simulink model "Working_TASS2_Fossen"  (Simulink 7.4)
settings: Solver=ode5  StartTime=0  StopTime=30  FixedStep=DeltaT  RelTol=1e-3
InitFcn:
  | %Bifocal Relay Mirror Spacecraft Dynamics Simulation          TA Sands
  | clear all;close all;clc;
  | 
  | %Constants0
  | Re=6371.2e3;mu=398601.2e9;          %earth radius and universal gravitation constant
  | 
  | %Spacecraft orbit
  | h=0;                                     %orbit altitude
  | R=Re+h;                             %orbit radius from center of earth
  | we=0.000072921158553;   %earth's angular velocity rad/solar sec(Vallado)
  | wo=sqrt(mu/(Re+h)^3);        %orbit angular velocity
  | incln=36.6001*pi/180;          %Inclination assumed Monterey Latitude
  | epsilon=12*pi/180;  alphao=0;
  | uo=0; nuo=0;                        %Start S/C beneath subsolar point
  | beta=60; gamma=1.5;
  | a=0.545491852; b=0.314939867;  c=0.704226952;   %Assumed spacecraft rectangular size
  | Area=[b*c a*c a*b];                 %projected area~m^2 in body x,y,z directions
  | density=4.39e-14;
  | kpre=-9.9639/24/3600/180*pi*0;      %nodal precession constant assumed zero here
  | wn=kpre*(Re/(Re+h))^3.5*cos(incln); %nodal precession (zero eccentricity)
  | V=wo*(Re+h);
  | rho=asin(Re/(h+Re));                %earth angular radius
  | Cd=2.5;     psun=4.5E-6;            %Drag coefficient and solar pressure constant~N/m^2
  | Kaero=-0.5*Cd*V^2;   Psolar=2*psun;  %constants for aero and solar torque calculation
  | dL=[0.002 0.002 0.008];             %predicted distance between cp and cg
  | Kme=2.3390e-005;
  | 
  | %Spacecraft Magnetic Properties (assumed)
  | mresid=[0 0 0.01];                  %Spacecraft residual magnetic moment
  | M=mresid;                           %Magnetic unit dipole vector
  | K=7.943e15;
  | 
  | %Spacecraft Inertia conditions
  | Ix=90;   Iy=100;   Iz=250 ;  % Ix=119.1259;   Iy=150.6615;   Iz=106.0288;;
  | Ixy=10;  Iyz=-20;  Ixz=10;   % Ixy=-15.7678;  Iyz=22.31637;  Ixz=-6.54859;
  | Imo=[Ix Ixy Ixz;
  |        Ixy  Iy  Iyz;
  |        Ixz Iyz  Iz];                  %Moment of inertia matrix
  | Iinv=inv(Imo);                      %Moment of inertia inverse goes in dynamics block
  | 
  | %Spacecraft initial Euler state angles and rates
  | phio=0;thetao=0;psio=0;                    %Initial Euler Angles
  | phidoto=0;thetadoto=0;psidoto=0;     %Initial Euler Rates
  | 
  | %Calculation of initial quaternion (qo) and angular momentum (Ho)
  | s1=sin(phio/2);s2=sin(thetao/2);s3=sin(psio/2);c1=cos(phio/2);c2=cos(thetao/2);c3=cos(psio/2);
  | q1o=s1*c2*c3-c1*s2*s3;
  | q2o=c1*s2*c3+s1*c2*s3;              %Wie pg. 321
  | q3o=c1*c2*s3-s1*s2*c3;
  | q4o=c1*c2*c3+s1*s2*s3;
  | S1=sin(phio);S2=sin(thetao);S3=sin(psio);C1=cos(phio);C2=cos(thetao);C3=cos(psio);
  | wxo=phidoto-psidoto*S2-wo*S3*C2;
  | wyo=thetadoto*C1+psidoto*C2*S1-wo*(C3*C1+S3*S2*S1);
  | wzo=psidoto*C2*C1-thetadoto*S1-wo*(S3*S2*C1-C3*S1);
  | qo=[q1o q2o q3o q4o];
  | Ho=Imo*[wxo wyo wzo]';
  | norm(Ho)*1000;
  | 
  | %Calculate eclipse time for comparison with EPS calculations
  | Te=100.87*2*V/2/pi;
  | 
  | %CMG Properties (in degrees)
  | %beta=90*pi/180;                                     %Skew angle in degrees converted to radians
  | beta=[90;90;-90;0]; beta=beta.*pi./180;
  | 
  | Gimbal0=[-30*pi/180; 90*pi/180; -30*pi/180;0];   % Initial Gimbal angles for 0 H spin up
  | w_wheel=2800*(2*pi/60);                       %Wheel speed in RPM converted to rad/s
  | Iwheel=0.0614*1.3558179483314;        % Wheel inertia in slug-ft^2 converted (exact) to kg m^2
  | h_wheel=Iwheel*w_wheel;                     % CMG Wheel Angular Momentum
  | 
  | %PID Controller Gains
  | %Kpx=2000;   Kdx=3250;   Kix=0;  Kpy=Kpx;   Kdy=Kdx;   Kiy=Kix;  Kpz=Kpx;   Kdz=Kdx;   Kiz=Kix;
  | Kpx=10100;   Kdx=1.6*Kpx;   Kix=0;  Kpy=Kpx;   Kdy=Kdx;   Kiy=Kix;  Kpz=Kpx;   Kdz=Kdx;   Kiz=Kix;
  | Kff=-1;
  | roll=0;  pitch=0; yaw=10;   roll=roll*pi/180; pitch=pitch*pi/180; yaw=yaw*pi/180;
  | SlewTime=10;  Rate=40;   DeltaT=1/Rate;   SPUDengage=0  %yaw*180/pi/100000
  | 
  | % [Fossen]'s adaptive feedforward parameters
  | ETA=1 ; LAMBDA=1;  ThetaHat0= [0;0;0;0;0;0;0;0;0];   ThetaHat0=[Ix; Ixy; Ixz; Iy; Iyz; Iz; 0; 0; 0];
StopFcn:
  | if flag==0; Hcmg=Hcmg;else;Hcmg=HcmgMP;end;
  | Hxcmg=[];Hycmg=[];Hzcmg=[];CondA=[]; CondA_MP=[];t=[]; SingPt=[];DetA=[];
  | for i=1:max(size(A));  t=[t i*DeltaT];  H=Hcmg(:,:,i); Hx=H(1,:);  Hy=H(2,:);  Hz=H(3,:);
  | detA=det(A(:,1:3,i));Hxcmg=[Hxcmg Hx];  Hycmg=[Hycmg Hy];  Hzcmg=[Hzcmg Hz];
  | CONDA=cond(A(:,:,i));  CONDA_MP=cond(A_MP(:,:,i));
  | DetA=[DetA detA]; CondA=[CondA CONDA];CondA_MP=[CondA_MP CONDA_MP];end;
  | Hmag=sqrt(Hxcmg.^2+Hycmg.^2+Hzcmg.^2);x=(max(t)-DeltaT);
  | 
  | if flag==0; MaxInvCond=min(1./CondA(10*Rate+1:end));DELTA=delta;DELTAdot=deltadot;
  | else; MaxInvCond=min(1./CondA_MP(10*Rate+1:end));DELTA=delta_MP;DELTAdot=deltadot_MP;Hcmg=HcmgMP;end;
  | ERROR=trajectory*180/pi-Euler;
  | 
  | %openfig('90_Degree_Singularity_Hypersurface');hold on;plot3(Hcmg(1,:),Hcmg(2,:),Hcmg(3,:), 'LineWidth',3);hold off;
  | 
  | figure(2);
  | subplot(2,1,1);plot(t,Hmag,'LineWidth',2);   ylabel('|H_c_m_g|','Fontsize',12);grid;axis([0,x,0,3]);
  | subplot(2,1,2);plot(t,DetA,'linewidth',2);grid;xlabel('t(sec)','fontsize',12,'fontname','times');ylabel('det[A]','fontsize',12,'fontname','times');axis([0,x,-1,1]);
  | 
  | 
  | DELTA1=DELTA(1,:);DELTA2=DELTA(2,:);DELTA3=DELTA(3,:);DELTA4=DELTA(4,:);
  | DELTAdot1=DELTAdot(1,:);DELTAdot2=DELTAdot(2,:);DELTAdot3=DELTAdot(3,:);DELTAdot4=DELTAdot(4,:);
  | 
  | figure(3);subplot(3,1,1);plot(t,DELTA1,'LineWidth',2); ylabel('\theta_1(deg)','Fontsize',12);grid;axis([0,x,min(DELTA1),max(DELTA1)]);
  | subplot(3,1,2);plot(t,DELTA2,'LineWidth',2); ylabel('\theta_2(deg)','Fontsize',12);grid;axis([0,x,min(DELTA2),max(DELTA2)])
  | subplot(3,1,3);plot(t,DELTA3,'LineWidth',2); ylabel('\theta_3(deg)','Fontsize',12);grid;axis([0,x,min(DELTA3),max(DELTA3)]);xlabel('t(sec)','Fontsize',12);
  | 
  | figure(4);subplot(3,1,1);plot(t,DELTAdot1,'LineWidth',2);   ylabel('\theta_d_o_t_1(deg/s)','Fontsize',12);grid;axis([0,x,-pi*1.1,pi*1.1])
  | subplot(3,1,2);plot(t,DELTAdot2,'LineWidth',2);   ylabel('\theta_d_o_t_2(deg/s)','Fontsize',12);grid;axis([0,x,-pi*1.1,pi*1.1])
  | subplot(3,1,3);plot(t,DELTAdot3,'LineWidth',2);   ylabel('\theta_d_o_t_3(deg/s)','Fontsize',12);grid;axis([0,x,-pi*1.1,pi*1.1]);xlabel('t(sec)','Fontsize',12);
  | 
  | figure(5);
  | subplot(3,1,1);plot(t,Hxcmg,'linewidth',2);axis([0,x,-3.25,3.25]);grid;ylabel('h_x/|h|','fontsize',14);title('Normalized Momentum','fontsize',14);
  | subplot(3,1,2);plot(t,Hycmg,'linewidth',2);axis([0,x,-3.25,3.25]);grid;ylabel('h_y/|h|','fontsize',14);
  | subplot(3,1,3);plot(t,Hzcmg,'linewidth',2);axis([0,x,-3.25,3.25]);grid;ylabel('h_z/|h|','fontsize',14);xlabel('t(sec)','fontsize',14);
  | 
  | figure(6); EulerX=Euler(:,1);EulerY=Euler(:,2);EulerZ=Euler(:,3);
  | subplot(3,1,1);plot(t,EulerX,'linewidth',2);  axis([0,x,-5,5]);          %axis([0,x,min(EulerX)*1.1,max(EulerX)*1.1]);
  |                        grid;ylabel('\phi(deg)','fontsize',16);title('Euler Angles','fontsize',14);
  | subplot(3,1,2);plot(t,EulerY,'linewidth',2);axis([0,x,-5,1.1*max(EulerY)]);  %axis([0,x,min(EulerY)*1.1,max(EulerY)*1.1]);
  |                         grid;ylabel('\theta(deg)','fontsize',16);
  | subplot(3,1,3);plot(t,EulerZ,'linewidth',2);axis([0,x,-5,1.1*max(EulerZ)]);  %axis([0,x,min(EulerZ)*1.1,max(EulerZ)*1.1]);
  |                         grid;ylabel('\psi(deg)','fontsize',16);xlabel('t(sec)','fontsize',14);
  | EX=ERROR(:,1);EY=ERROR(:,2);EZ=ERROR(:,3);
  | MeanXerror=mean(EX); Xmean=num2str(MeanXerror); xmean=['\mu_x=', Xmean];
  | STDx=std(EX);Xsigma=num2str(STDx);SigmaX=['\sigma_x=' Xsigma];
  | MeanYerror=mean(EY); Ymean=num2str(MeanYerror); ymean=['\mu_y=', Ymean];
  | STDy=std(EY); Ysigma=num2str(STDy);SigmaY=['\sigma_y=' Ysigma];
  | MeanZerror=mean(EZ); Zmean=num2str(MeanZerror); zmean=['\mu_z=', Zmean];
  | STDz=std(EZ);Zsigma=num2str(STDz);SigmaZ=['\sigma_z=' Zsigma];
  | MeanError=[MeanXerror MeanYerror MeanZerror];  StdDev=[STDx STDy STDz];
  | 
  | figure(7);
  | subplot(3,1,1);plot(t,EX,'linewidth',2);axis([0,x,-5,5]);  % axis([0,x,min(EX)*1.1,max(EX)*1.1]);
  |   grid;ylabel('\phi(deg)','fontsize',16);title('Tracking Error','fontsize',14);
  |   text(x*2/3,max(EX)*2/3,xmean,'fontsize',12,'fontname','times');  text(x*2/3,max(EX)*1/3,SigmaX,'fontsize',12,'fontname','times');
  | subplot(3,1,2);plot(t,EY,'linewidth',2);axis([0,x,-5,5]);  %axis([0,x,min(EY)*1.1,max(EY)*1.1]);
  |   grid;ylabel('\theta(deg)','fontsize',16);
  |   text(x*2/3,min(EY)*2/3,ymean,'fontsize',12,'fontname','times');  text(x*2/3,min(EY)*1/3,SigmaY,'fontsize',12,'fontname','times');
  | subplot(3,1,3);plot(t,EZ,'linewidth',2);axis([0,x,-5,5]);  %axis([0,x,min(EZ)*1.1,max(EZ)*1.1]);
  |   grid;ylabel('\psi(deg)','fontsize',16);xlabel('t(sec)','fontsize',14);
  |   text(x*2/3,max(EZ)*2/3,zmean,'fontsize',12,'fontname','times');  text(x*2/3,max(EZ)*1/3,SigmaZ,'fontsize',12,'fontname','times');
  | 
  | figure(8);subplot(3,3,1);plot(t,THETAhat(:,1));grid; axis([0,max(t), min(THETAhat(:,1)),max(THETAhat(:,1))]);
  | subplot(3,3,2);plot(t,THETAhat(:,2));grid;axis([0,max(t), min(THETAhat(:,2)),max(THETAhat(:,2))]);
  | subplot(3,3,3);plot(t,THETAhat(:,3));grid;axis([0,max(t), min(THETAhat(:,3)),max(THETAhat(:,3))]);
  | subplot(3,3,4);plot(t,THETAhat(:,2));grid;axis([0,max(t), min(THETAhat(:,2)),max(THETAhat(:,2))]);
  | subplot(3,3,5);plot(t,THETAhat(:,4));grid;axis([0,max(t), min(THETAhat(:,4)),max(THETAhat(:,4))]);
  | subplot(3,3,6);plot(t,THETAhat(:,5));grid;axis([0,max(t), min(THETAhat(:,5)),max(THETAhat(:,5))]);
  | subplot(3,3,7);plot(t,THETAhat(:,3));grid;axis([0,max(t), min(THETAhat(:,3)),max(THETAhat(:,3))]);
  | subplot(3,3,8);plot(t,THETAhat(:,5));grid;axis([0,max(t), min(THETAhat(:,5)),max(THETAhat(:,5))]);
  | subplot(3,3,9);plot(t,THETAhat(:,6));grid;axis([0,max(t), min(THETAhat(:,6)),max(THETAhat(:,6))]);
  | 
  | figure(9);subplot(2,1,1);plot(t,ufb,'linewidth',2);grid;
  |   m1=min(ufb(:,1));m2=min(ufb(:,2));m3=min(ufb(:,3)); m=[m1,m2,m3];
  |   M1=max(ufb(:,1));M2=max(ufb(:,2));M3=max(ufb(:,3)); M=[M1,M2,M3];
  |   axis([0, max(t),min(m),max(M)]);
  |   ylabel('Feedback Control','fontname','times','fontsize',14);
  |   legend('\phi','\theta','\psi','Location','SouthEast');
  | subplot(2,1,2);plot(t,uff,'linewidth',2);grid;
  |   m1=min(uff(:,1));m2=min(uff(:,2));m3=min(uff(:,3)); m=[m1,m2,m3];
  |   M1=max(uff(:,1));M2=max(uff(:,2));M3=max(uff(:,3)); M=[M1,M2,M3];
  |   axis([0, max(t),min(m),max(M)]);
  |   legend('\phi','\theta','\psi','Location','NorthEast');
  |   ylabel('FeedForward Control','fontname','times','fontsize',14);      xlabel('time(sec)','fontname','times','fontsize',14)
  | Jhat=[THETAhat(end,1)  THETAhat(end,2) THETAhat(end,3); THETAhat(end,2) THETAhat(end,4) THETAhat(end,5); THETAhat(end,3) THETAhat(end,5) THETAhat(end,6)]
  | Imo
undefined symbols (not defined in the file): svd
libraries: aerospace x4, simulink x4, simulink_extras x3, dspinverses x2
settings Model: Creator=tasands  LastModifiedBy=tasands
settings DataIOCC: SignalLoggingName=sigsOut
settings OptimizationCC: InlineInvariantSignals=on  InitFltsAndDblsToZero=on
settings DebuggingCC: SaveWithParameterizedLinksMsg=none  SignalResolutionControl=TryResolveAllWithWarning  SolverPrmCheckMsg=none  MultiTaskDSMMsg=warning  MultiTaskCondExecSysMsg=none  StrictBusMsg=None
settings HardwareCC: TargetHWDeviceType=32-bit Generic  ProdEqTarget=off
settings RTWCC: IncludeERTFirstTime=on
settings GRTTargetCC: TargetFcnLib=ansi_tfl_tmw.mat

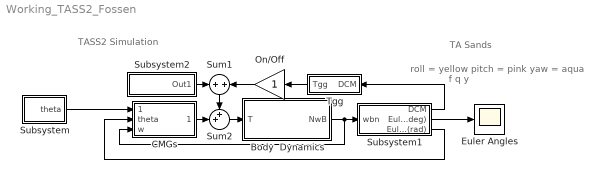
== system Working_TASS2_Fossen ==
  note: roll = yellow
      | pitch = pink
      | yaw = aqua
  note: TASS2 Simulation
  note: TA Sands
  note: f
      | q
      | y
  Body  Dynamics : Subsystem
      mask Display: disp('TASS2 Dynamics')
  CMGs : Subsystem
      mask Display: disp('Control')
  Euler Angles : Scope
      settings: TimeRange=30  YMin=-100  YMax=100
  On/Off : Gain  ParameterDataType=sfix(16)  ParameterScaling=2^0  OutDataType=sfix(16)  OutScaling=2^0  SaturateOnIntegerOverflow=on  OutDataTypeStr=Inherit: Same as input  ParamDataTypeStr=Inherit: Same as input
  Subsystem : Subsystem
      mask Display: disp('Slew')
  Subsystem1 : Subsystem
      mask Display: disp('Kinematics')
  Subsystem2 : Subsystem
      mask Display: disp('Disturbances')
  Sum1 : Sum  OutDataType=sfix(16)  OutScaling=2^0  SaturateOnIntegerOverflow=on
  Sum2 : Sum  Inputs=++|  OutDataType=sfix(16)  OutScaling=2^0  SaturateOnIntegerOverflow=on
  Tgg : Subsystem
      mask Display: disp('CG offet')
  wires:
  Sum2/1 -> Body  Dynamics/1(T)
  Body  Dynamics/1(NwB) -> Subsystem1/1(wbn), CMGs/3(w)
  CMGs/1(Tactual) -> Sum2/2
  Sum1/1 -> Sum2/1
  Subsystem2/1(Out1) -> Sum1/1
  Tgg/1(Tgg) -> On/Off/1
  Subsystem/1(theta) -> CMGs/1(ThetaCMD)
  Subsystem1/1(DCM) -> Tgg/1(DCM)
  Subsystem1/2(Euler(deg)) -> Euler Angles/1
  Subsystem1/3(Euler(rad)) -> CMGs/2(theta)
  On/Off/1 -> Sum1/2

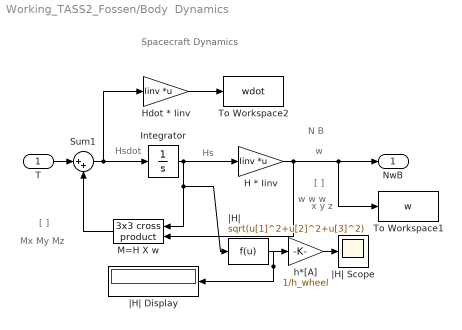
== system Working_TASS2_Fossen/Body  Dynamics ==
  note: w
  note: N B
  note: Hs
  note: Hsdot
  note: [ ]
  note: Mx
      | My
      | Mz
  note: [ ]
  note: w
      | w
      | w
  note: x
      | y
      | z
  note: Spacecraft Dynamics
  T : Inport  OutDataType=sfix(16)  OutScaling=2^0
  H * Iinv : Gain  Gain=Iinv  Multiplication=Matrix(K*u)  ParameterDataType=sfix(16)  ParameterScaling=2^0  OutDataType=sfix(16)  OutScaling=2^0  SaturateOnIntegerOverflow=on  OutDataTypeStr=Inherit: Same as input  ParamDataTypeStr=Inherit: Same as input
  Hdot * Iinv : Gain  Gain=Iinv  Multiplication=Matrix(K*u)  ParameterDataType=sfix(16)  ParameterScaling=2^0  OutDataType=sfix(16)  OutScaling=2^0  SaturateOnIntegerOverflow=on  OutDataTypeStr=Inherit: Same as input  ParamDataTypeStr=Inherit: Same as input
  Integrator : Integrator
  M=H X w : aerospace/Axes Transformations/3x3 cross product  SystemSampleTime=-1
  Sum1 : Sum  Inputs=|++  OutDataType=sfix(16)  OutScaling=2^0  SaturateOnIntegerOverflow=on  InputSameDT=on  OutDataTypeStr=Inherit: Same as first input
  To Workspace1 : ToWorkspace  VariableName=w  SampleTime=-1  SaveFormat=Array
  To Workspace2 : ToWorkspace  VariableName=wdot  SampleTime=-1  SaveFormat=Array
  h*[A] : Gain  Gain=1/h_wheel  ParameterDataType=sfix(16)  ParameterScaling=2^0  OutDataType=sfix(16)  OutScaling=2^0
  |H| : Fcn  Expr=sqrt(u[1]^2+u[2]^2+u[3]^2)
  |H| Display : Display
  |H| Scope : Scope
      settings: TimeRange=30  YMin=0  YMax=1.4
  NwB : Outport  OutDataType=sfix(16)  OutScaling=2^0
  wires:
  Integrator/1 -> H * Iinv/1, M=H X w/1, |H|/1
  H * Iinv/1 -> M=H X w/2, NwB/1, To Workspace1/1
  M=H X w/1 -> Sum1/2
  |H|/1 -> |H| Display/1, h*[A]/1
  Sum1/1 -> Integrator/1, Hdot * Iinv/1
  T/1 -> Sum1/1
  h*[A]/1 -> |H| Scope/1
  Hdot * Iinv/1 -> To Workspace2/1

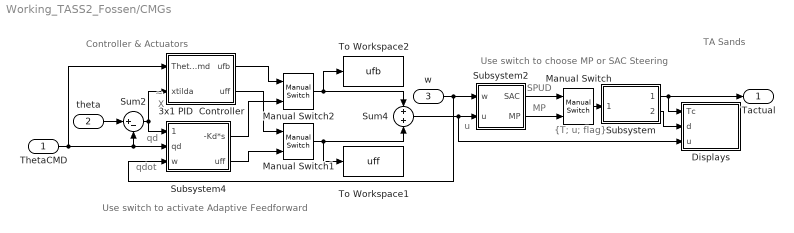
== system Working_TASS2_Fossen/CMGs ==
  note: Use switch to choose
      | MP or SAC Steering
  note: u
  note: SPUD
  note: MP
  note: {T; u; flag}
  note: TA Sands
  note: Controller & Actuators
  note: X
  note: ~
  note: qd
  note: Use switch to activate
      | Adaptive Feedforward
  note: qdot
  ThetaCMD : Inport  OutDataType=sfix(16)  OutScaling=2^0
  theta : Inport  Port=2  OutDataType=sfix(16)  OutScaling=2^0
  w : Inport  Port=3  OutDataType=sfix(16)  OutScaling=2^0
  3x1 PID  Controller : Subsystem
      mask Display: disp('Classical')
  Displays : Subsystem
      mask Display: disp('Displays')
  Manual Switch : simulink/Signal Routing/Manual Switch  SystemSampleTime=-1  sw=1  action=0  varsize=off
  Manual Switch1 : simulink/Signal Routing/Manual Switch  SystemSampleTime=-1  sw=0  action=0  varsize=off
  Manual Switch2 : simulink/Signal Routing/Manual Switch  SystemSampleTime=-1  sw=0  action=0  varsize=off
  Subsystem : Subsystem
      mask Display: disp('DeMux')
  Subsystem2 : Subsystem
      mask Display: disp('CMGs')
  Subsystem4 : Subsystem
      mask Display: disp('[Fossen]')
  Sum2 : Sum  Inputs=|+-  OutDataType=sfix(16)  OutScaling=2^0  SaturateOnIntegerOverflow=on
  Sum4 : Sum  OutDataType=sfix(16)  OutScaling=2^0  SaturateOnIntegerOverflow=on
  To Workspace1 : ToWorkspace  VariableName=uff  SampleTime=-1  SaveFormat=Array
  To Workspace2 : ToWorkspace  VariableName=ufb  SampleTime=-1  SaveFormat=Array
  Tactual : Outport  OutDataType=sfix(16)  OutScaling=2^0
  wires:
  theta/1 -> Sum2/1
  Sum2/1 -> 3x1 PID  Controller/2(xtilda), Subsystem4/1(LAMBDA*xtilda)
  ThetaCMD/1 -> Sum2/2, Subsystem4/2(qd), 3x1 PID  Controller/1(ThetaCmd)
  Subsystem/1(Torque) -> Displays/1(Tc), Tactual/1
  Subsystem/2(GimbalAngles) -> Displays/2(d)
  w/1 -> Subsystem2/1(w), Subsystem4/3(w)
  Subsystem2/1(SAC) -> Manual Switch/1
  Subsystem2/2(MP) -> Manual Switch/2
  Manual Switch/1 -> Subsystem/1(SAC/MP)
  3x1 PID  Controller/1(ufb) -> Manual Switch2/1
  Subsystem4/1(-Kd*s) -> Manual Switch2/2
  3x1 PID  Controller/2(uff) -> Manual Switch1/1
  Subsystem4/2(uff) -> Manual Switch1/2
  Manual Switch2/1 -> Sum4/1, To Workspace2/1
  Manual Switch1/1 -> Sum4/2, To Workspace1/1
  Sum4/1 -> Subsystem2/2(u), Displays/3(u)

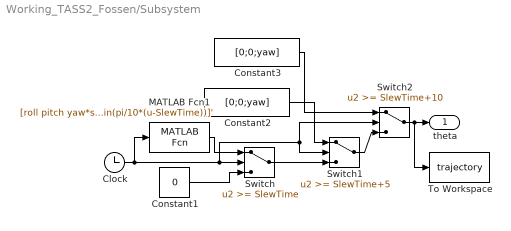
== system Working_TASS2_Fossen/Subsystem ==
  Clock : Clock
      settings: Decimation=10
  Constant1 : Constant  Value=0  OutDataType=sfix(16)  OutScaling=2^0
  Constant2 : Constant  Value=[0;0;yaw]  OutDataType=sfix(16)  OutScaling=2^0
  Constant3 : Constant  Value=[0;0;yaw]  OutDataType=sfix(16)  OutScaling=2^0
  MATLAB Fcn1 : MATLABFcn  MATLABFcn=[roll pitch yaw*sin(pi/10*(u-SlewTime))]'
  Switch : Switch  Threshold=SlewTime
  Switch1 : Switch  Threshold=SlewTime+5
  Switch2 : Switch  Threshold=SlewTime+10
  To Workspace : ToWorkspace  VariableName=trajectory  SampleTime=-1  SaveFormat=Array
  theta : Outport  OutDataType=sfix(16)  OutScaling=2^0
  wires:
  Constant3/1 -> Switch2/1
  Switch1/1 -> Switch2/3
  Switch/1 -> Switch1/3
  Constant1/1 -> Switch/3
  Clock/1 -> Switch/2, Switch1/2, Switch2/2, MATLAB Fcn1/1
  MATLAB Fcn1/1 -> Switch/1
  Constant2/1 -> Switch1/1
  Switch2/1 -> theta/1, To Workspace/1

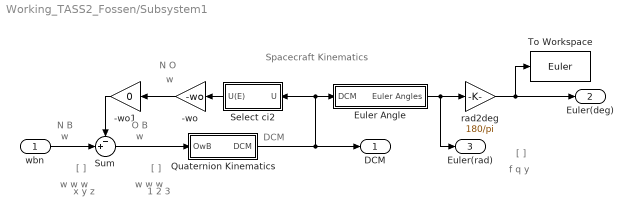
== system Working_TASS2_Fossen/Subsystem1 ==
  note: [ ]
  note: w
      | w
      | w
  note: x
      | y
      | z
  note: w
  note: N B
  note: w
  note: [ ]
  note: w
      | w
      | w
  note: 1
      | 2
      | 3
  note: w
  note: O B
  note: DCM
  note: N O
  note: [ ]
  note: f
      | q
      | y
  note: Spacecraft Kinematics
  wbn : Inport  OutDataType=sfix(16)  OutScaling=2^0
  -wo : Gain  Gain=-wo  ParameterDataType=sfix(16)  ParameterScaling=2^0  OutDataType=sfix(16)  OutScaling=2^0  SaturateOnIntegerOverflow=on  OutDataTypeStr=Inherit: Same as input  ParamDataTypeStr=Inherit: Same as input
  -wo1 : Gain  Gain=0  ParameterDataType=sfix(16)  ParameterScaling=2^0  OutDataType=sfix(16)  OutScaling=2^0  SaturateOnIntegerOverflow=on  OutDataTypeStr=Inherit: Same as input  ParamDataTypeStr=Inherit: Same as input
  Euler Angle : Subsystem
  Quaternion Kinematics : Subsystem
  Select ci2 : Subsystem
  Sum : Sum  Inputs=-+|  OutDataType=sfix(16)  OutScaling=2^0  SaturateOnIntegerOverflow=on  InputSameDT=on  OutDataTypeStr=Inherit: Same as first input
  To Workspace : ToWorkspace  VariableName=Euler  SampleTime=-1  SaveFormat=Array
  rad2deg : Gain  Gain=180/pi  ParameterDataType=sfix(16)  ParameterScaling=2^0  OutDataType=sfix(16)  OutScaling=2^0  SaturateOnIntegerOverflow=on  OutDataTypeStr=Inherit: Same as input  ParamDataTypeStr=Inherit: Same as input
  DCM : Outport  OutDataType=sfix(16)  OutScaling=2^0
  Euler(deg) : Outport  Port=2  OutDataType=sfix(16)  OutScaling=2^0
  Euler(rad) : Outport  Port=3  OutDataType=sfix(16)  OutScaling=2^0
  wires:
  Sum/1 -> Quaternion Kinematics/1(OwB)
  -wo/1 -> -wo1/1
  Select ci2/1(U(E)) -> -wo/1
  Quaternion Kinematics/1(DCM) -> Select ci2/1(U), Euler Angle/1(DCM), DCM/1
  -wo1/1 -> Sum/1
  wbn/1 -> Sum/2
  Euler Angle/1(Euler Angles) -> rad2deg/1, Euler(rad)/1
  rad2deg/1 -> Euler(deg)/1, To Workspace/1

== system Working_TASS2_Fossen/Subsystem2 ==
  Tdisturbance : Step  Time=0  After=0  SampleTime=0
  Out1 : Outport  OutDataType=sfix(16)  OutScaling=2^0
  wires:
  Tdisturbance/1 -> Out1/1

== system Working_TASS2_Fossen/Tgg ==
  note: Gravity Gradient Torques
  DCM : Inport  OutDataType=sfix(16)  OutScaling=2^0
  3*mu/Ro^3 : Gain  Gain=3*mu/(h+Re)^3  Multiplication=Matrix(K*u)  ParameterDataType=sfix(16)  ParameterScaling=2^0  OutDataType=sfix(16)  OutScaling=2^0  SaturateOnIntegerOverflow=on  OutDataTypeStr=Inherit: Same as input  ParamDataTypeStr=Inherit: Same as input
  3x3 cross product : aerospace/Axes Transformations/3x3 cross product  SystemSampleTime=-1
  Jbody : Gain  Gain=Imo  Multiplication=Matrix(K*u)  ParameterDataType=sfix(16)  ParameterScaling=2^0  OutDataType=sfix(16)  OutScaling=2^0  SaturateOnIntegerOverflow=on  OutDataTypeStr=Inherit: Same as input  ParamDataTypeStr=Inherit: Same as input
  On/Off : Gain  ParameterDataType=sfix(16)  ParameterScaling=2^0  OutDataType=sfix(16)  OutScaling=2^0  SaturateOnIntegerOverflow=on  OutDataTypeStr=Inherit: Same as input  ParamDataTypeStr=Inherit: Same as input
  Select ci3 : Subsystem
  Tgg : Outport  OutDataType=sfix(16)  OutScaling=2^0
  wires:
  Jbody/1 -> 3x3 cross product/2
  3*mu/Ro^3/1 -> On/Off/1
  3x3 cross product/1 -> 3*mu/Ro^3/1
  Select ci3/1(U(E)) -> 3x3 cross product/1, Jbody/1
  DCM/1 -> Select ci3/1(U)
  On/Off/1 -> Tgg/1

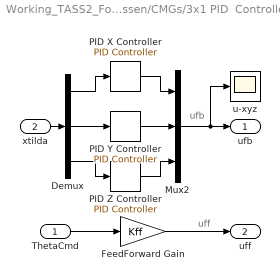
== system Working_TASS2_Fossen/CMGs/3x1 PID  Controller ==
  note: ufb
  note: uff
  ThetaCmd : Inport  OutDataType=sfix(16)  OutScaling=2^0
  xtilda : Inport  Port=2  OutDataType=sfix(16)  OutScaling=2^0
  Demux : Demux  Outputs=3
  FeedForward Gain : Gain  Gain=Kff  ParameterDataType=sfix(16)  ParameterScaling=2^0  OutDataType=sfix(16)  OutScaling=2^0  SaturateOnIntegerOverflow=on  OutDataTypeStr=Inherit: Same as input  ParamDataTypeStr=Inherit: Same as input
  Mux2 : Mux  Inputs=3
  PID X Controller : simulink_extras/Additional Linear/PID Controller  SystemSampleTime=-1  P=Kpx  I=Kix  D=Kdx
  PID Y Controller : simulink_extras/Additional Linear/PID Controller  SystemSampleTime=-1  P=Kpy  I=Kiy  D=Kdy
  PID Z Controller : simulink_extras/Additional Linear/PID Controller  SystemSampleTime=-1  P=Kpz  I=Kiz  D=Kdz
  u-xyz : Scope
      settings: TimeRange=120  YMin=-100  YMax=150  SaveName=ScopeData3
  ufb : Outport  OutDataType=sfix(16)  OutScaling=2^0
  uff : Outport  Port=2  OutDataType=sfix(16)  OutScaling=2^0
  wires:
  xtilda/1 -> Demux/1
  Demux/1 -> PID X Controller/1
  Demux/2 -> PID Y Controller/1
  Demux/3 -> PID Z Controller/1
  PID X Controller/1 -> Mux2/1
  PID Y Controller/1 -> Mux2/2
  PID Z Controller/1 -> Mux2/3
  Mux2/1 -> ufb/1, u-xyz/1
  ThetaCmd/1 -> FeedForward Gain/1
  FeedForward Gain/1 -> uff/1

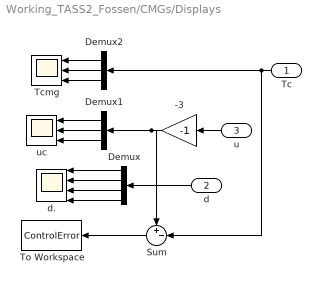
== system Working_TASS2_Fossen/CMGs/Displays ==
  Tc : Inport  OutDataType=sfix(16)  OutScaling=2^0
  d : Inport  Port=2  OutDataType=sfix(16)  OutScaling=2^0
  u : Inport  Port=3  OutDataType=sfix(16)  OutScaling=2^0
  -3 : Gain  Gain=-1  ParameterDataType=sfix(16)  ParameterScaling=2^0  OutDataType=sfix(16)  OutScaling=2^0  SaturateOnIntegerOverflow=on  OutDataTypeStr=Inherit: Same as input  ParamDataTypeStr=Inherit: Same as input
  Demux : Demux
  Demux1 : Demux  Outputs=3
  Demux2 : Demux  Outputs=3
  Sum : Sum  Inputs=+-|  OutDataType=sfix(16)  OutScaling=2^0
  Tcmg : Scope  NumInputPorts=3
      settings: TimeRange=30  YMin=-50~-100~-200  YMax=50~100~200  SaveName=ScopeData7
  To Workspace : ToWorkspace  VariableName=ControlError  SampleTime=-1  SaveFormat=Array
  d. : Scope  NumInputPorts=4
      settings: TimeRange=30  YMin=-200~-80~-300~-1  YMax=400~0~100~1  SaveName=ScopeData2
  uc : Scope  NumInputPorts=3
      settings: TimeRange=30  YMin=-50~-1000~-50000  YMax=50~1000~50000  SaveName=ScopeData6
  wires:
  d/1 -> Demux/1
  u/1 -> -3/1
  Demux/4 -> d./4
  Demux/3 -> d./3
  Demux/2 -> d./2
  Demux/1 -> d./1
  -3/1 -> Demux1/1, Sum/1
  Tc/1 -> Demux2/1, Sum/2
  Demux2/1 -> Tcmg/1
  Demux2/2 -> Tcmg/2
  Demux2/3 -> Tcmg/3
  Demux1/1 -> uc/1
  Demux1/2 -> uc/2
  Demux1/3 -> uc/3
  Sum/1 -> To Workspace/1

== system Working_TASS2_Fossen/CMGs/Subsystem ==
  SAC/MP : Inport  OutDataType=sfix(16)  OutScaling=2^0
  Demux : Demux  Outputs=8
  Mux : Mux  Inputs=3
  Mux1 : Mux
  To Workspace : ToWorkspace  VariableName=flag  SampleTime=-1  SaveFormat=Array
  Torque : Outport  OutDataType=sfix(16)  OutScaling=2^0
  GimbalAngles : Outport  Port=2  OutDataType=sfix(16)  OutScaling=2^0
  wires:
  SAC/MP/1 -> Demux/1
  Demux/8 -> To Workspace/1
  Demux/1 -> Mux/1
  Demux/2 -> Mux/2
  Demux/3 -> Mux/3
  Demux/4 -> Mux1/1
  Demux/5 -> Mux1/2
  Demux/6 -> Mux1/3
  Demux/7 -> Mux1/4
  Mux1/1 -> GimbalAngles/1
  Mux/1 -> Torque/1

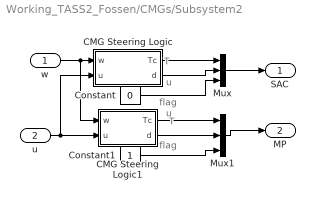
== system Working_TASS2_Fossen/CMGs/Subsystem2 ==
  note: flag
  note: flag
  note: u
  note: T
  note: u
  note: T
  w : Inport  OutDataType=sfix(16)  OutScaling=2^0
  u : Inport  Port=2  OutDataType=sfix(16)  OutScaling=2^0
  CMG Steering Logic : Subsystem
      mask Display: disp('SPUD Steer')
  CMG Steering Logic1 : Subsystem
      mask Display: disp('MP Steer')
  Constant : Constant  Value=0  OutDataType=sfix(16)  OutScaling=2^0
  Constant1 : Constant  OutDataType=sfix(16)  OutScaling=2^0
  Mux : Mux  Inputs=3
  Mux1 : Mux  Inputs=3
  SAC : Outport  OutDataType=sfix(16)  OutScaling=2^0
  MP : Outport  Port=2  OutDataType=sfix(16)  OutScaling=2^0
  wires:
  u/1 -> CMG Steering Logic1/2(u), CMG Steering Logic/2(u)
  Mux1/1 -> MP/1
  Mux/1 -> SAC/1
  Constant1/1 -> Mux1/3
  Constant/1 -> Mux/3
  CMG Steering Logic1/2(d) -> Mux1/2
  CMG Steering Logic1/1(Tc) -> Mux1/1
  CMG Steering Logic/2(d) -> Mux/2
  CMG Steering Logic/1(Tc) -> Mux/1
  w/1 -> CMG Steering Logic1/1(w), CMG Steering Logic/1(w)

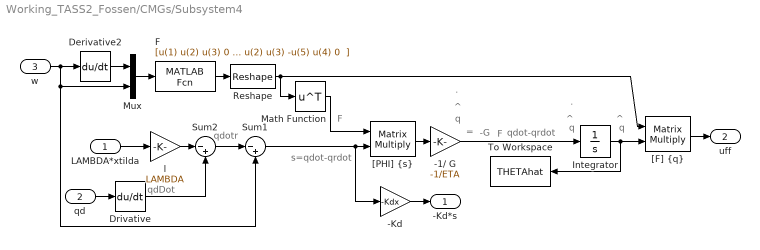
== system Working_TASS2_Fossen/CMGs/Subsystem4 ==
  note: qdotr
  note: s=qdot-qrdot
  note: qdDot
  note: q
  note: ^
  note: F
  note: -G
  note: F
  note: =
  note: ^
  note: q
  note: ^
  note: q
  note: .
  note: .
  note: qdot-qrdot
  LAMBDA*xtilda : Inport  OutDataType=sfix(16)  OutScaling=2^0
  qd : Inport  Port=2  OutDataType=sfix(16)  OutScaling=2^0
  w : Inport  Port=3  OutDataType=sfix(16)  OutScaling=2^0
  -1/ G : Gain  Gain=-1/ETA  ParameterDataType=sfix(16)  ParameterScaling=2^0  OutDataType=sfix(16)  OutScaling=2^0  SaturateOnIntegerOverflow=on  OutDataTypeStr=Inherit: Same as input  ParamDataTypeStr=Inherit: Same as input
  -Kd : Gain  Gain=-Kdx  ParameterDataType=sfix(16)  ParameterScaling=2^0  OutDataType=sfix(16)  OutScaling=2^0  SaturateOnIntegerOverflow=on  OutDataTypeStr=Inherit: Same as input  ParamDataTypeStr=Inherit: Same as input
  Derivative2 : Derivative
  Drivative : Derivative
  F : MATLABFcn  MATLABFcn="[u(1) u(2) u(3) 0 0 0 0 -u(6) u(5);  0 u(1) 0 u(2) u(3) 0 u(6) 0 u(4);  0 0 u(1) 0 u(2) u(3) -u(5) u(4) 0  ]"
  Integrator : Integrator  InitialCondition=ThetaHat0
  Math Function : Math  Operator=transpose  OutDataType=sfix(16)  OutScaling=2^0  SaturateOnIntegerOverflow=on
  Mux : Mux  Inputs=2
  Reshape : Reshape  OutputDimensionality=Customize  OutputDimensions=[3,9]
  Sum1 : Sum  Inputs=|-+  OutDataType=sfix(16)  OutScaling=2^0  SaturateOnIntegerOverflow=on
  Sum2 : Sum  Inputs=|-+  OutDataType=sfix(16)  OutScaling=2^0  SaturateOnIntegerOverflow=on
  To Workspace : ToWorkspace  VariableName=THETAhat  SampleTime=-1  SaveFormat=Array
  "[F] {q}" : Product  Multiplication=Matrix(*)  OutDataType=sfix(16)  OutScaling=2^0  SaturateOnIntegerOverflow=on  OutDataTypeStr=Inherit: Same as first input
  "[PHI] {s}" : Product  Multiplication=Matrix(*)  OutDataType=sfix(16)  OutScaling=2^0  SaturateOnIntegerOverflow=on  OutDataTypeStr=Inherit: Same as first input
  l : Gain  Gain=LAMBDA  ParameterDataType=sfix(16)  ParameterScaling=2^0  OutDataType=sfix(16)  OutScaling=2^0  SaturateOnIntegerOverflow=on  OutDataTypeStr=Inherit: Same as input  ParamDataTypeStr=Inherit: Same as input
  -Kd*s : Outport  OutDataType=sfix(16)  OutScaling=2^0
  uff : Outport  Port=2  OutDataType=sfix(16)  OutScaling=2^0
  wires:
  LAMBDA*xtilda/1 -> l/1
  l/1 -> Sum2/1
  Sum2/1 -> Sum1/1
  Sum1/1 -> "[PHI] {s}"/2, -Kd/1
  "[PHI] {s}"/1 -> -1/ G/1
  F/1 -> Reshape/1
  qd/1 -> Drivative/1
  Drivative/1 -> Sum2/2
  w/1 -> Derivative2/1, Sum1/2, Mux/2
  Mux/1 -> F/1
  Derivative2/1 -> Mux/1
  -1/ G/1 -> Integrator/1
  Integrator/1 -> "[F] {q}"/2, To Workspace/1
  Math Function/1 -> "[PHI] {s}"/1
  Reshape/1 -> "[F] {q}"/1, Math Function/1
  "[F] {q}"/1 -> uff/1
  -Kd/1 -> -Kd*s/1

== system Working_TASS2_Fossen/Subsystem1/Euler Angle ==
  note: q
  note: f
  note: y
  note: q
  DCM : Inport  OutDataType=sfix(16)  OutScaling=2^0
  -asin(C13) : Fcn  Expr=-asin(u[3])
  C12 : Fcn  Expr=u[2]
  C23 : Fcn  Expr=u[6]
  Fcn : Fcn  Expr="asin(u[2]/cos(u[1])  )"
  Fcn1 : Fcn  Expr=asin(u[1]/cos(u[2]))
  Mux : Mux  Inputs=3
  Mux1 : Mux  Inputs=2
  Mux2 : Mux  Inputs=2
  Euler Angles : Outport  OutDataType=sfix(16)  OutScaling=2^0
  wires:
  C12/1 -> Mux2/2
  Fcn/1 -> Mux/3
  Mux2/1 -> Fcn/1
  C23/1 -> Mux1/1
  -asin(C13)/1 -> Mux2/1, Mux1/2, Mux/2
  Fcn1/1 -> Mux/1
  Mux1/1 -> Fcn1/1
  DCM/1 -> C12/1, C23/1, -asin(C13)/1
  Mux/1 -> Euler Angles/1

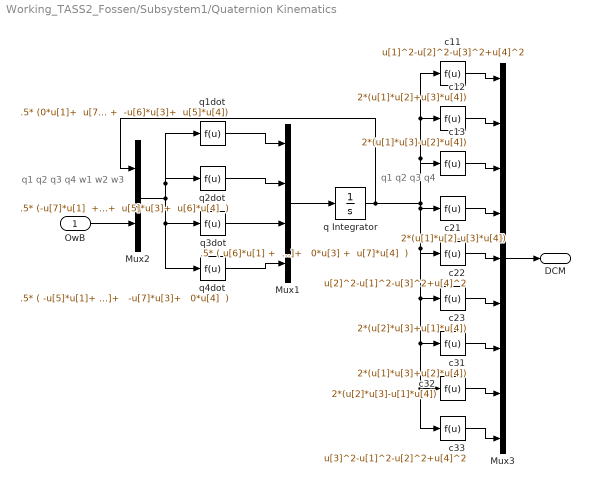
== system Working_TASS2_Fossen/Subsystem1/Quaternion Kinematics ==
  note: q1
      | q2
      | q3
      | q4
      | w1
      | w2
      | w3
  note: q1
      | q2
      | q3
      | q4
  OwB : Inport  OutDataType=sfix(16)  OutScaling=2^0
  Mux1 : Mux
  Mux2 : Mux  Inputs=2
  Mux3 : Mux  Inputs=9
  c11 : Fcn  Expr=u[1]^2-u[2]^2-u[3]^2+u[4]^2
  c12 : Fcn  Expr=2*(u[1]*u[2]+u[3]*u[4])
  c13 : Fcn  Expr=2*(u[1]*u[3]-u[2]*u[4])
  c21 : Fcn  Expr=2*(u[1]*u[2]-u[3]*u[4])
  c22 : Fcn  Expr=u[2]^2-u[1]^2-u[3]^2+u[4]^2
  c23 : Fcn  Expr=2*(u[2]*u[3]+u[1]*u[4])
  c31 : Fcn  Expr=2*(u[1]*u[3]+u[2]*u[4])
  c32 : Fcn  Expr=2*(u[2]*u[3]-u[1]*u[4])
  c33 : Fcn  Expr=u[3]^2-u[1]^2-u[2]^2+u[4]^2
  q Integrator : Integrator  InitialCondition=qo
  q1dot : Fcn  Expr=".5* (0*u[1]+  u[7]*u[2] +  -u[6]*u[3]+  u[5]*u[4])"
  q2dot : Fcn  Expr=".5* (-u[7]*u[1]  +  0*u[2]+  u[5]*u[3]+  u[6]*u[4]  )"
  q3dot : Fcn  Expr=".5* ( u[6]*u[1] +  -u[5]*u[2]+   0*u[3] +  u[7]*u[4]  )"
  q4dot : Fcn  Expr=".5* ( -u[5]*u[1]+   -u[6]*u[2]+   -u[7]*u[3]+   0*u[4]  )"
  DCM : Outport  OutDataType=sfix(16)  OutScaling=2^0
  wires:
  OwB/1 -> Mux2/2
  q1dot/1 -> Mux1/1
  q2dot/1 -> Mux1/2
  q3dot/1 -> Mux1/3
  q4dot/1 -> Mux1/4
  Mux1/1 -> q Integrator/1
  q Integrator/1 -> c13/1, c12/1, c11/1, c21/1, c22/1, c23/1, c31/1, c33/1, c32/1, Mux2/1
  c11/1 -> Mux3/1
  c12/1 -> Mux3/2
  c13/1 -> Mux3/3
  c22/1 -> Mux3/5
  c21/1 -> Mux3/4
  c23/1 -> Mux3/6
  c31/1 -> Mux3/7
  c32/1 -> Mux3/8
  c33/1 -> Mux3/9
  Mux3/1 -> DCM/1
  Mux2/1 -> q2dot/1, q1dot/1, q3dot/1, q4dot/1

== system Working_TASS2_Fossen/Subsystem1/Select ci2 ==
  U : Inport  OutDataType=sfix(16)  OutScaling=2^0
  C12 : Fcn  Expr=u[2]
  C22 : Fcn  Expr=u[5]
  C32 : Fcn  Expr=u[8]
  Mux2 : Mux  Inputs=3
  U(E) : Outport  OutDataType=sfix(16)  OutScaling=2^0
  wires:
  C12/1 -> Mux2/1
  C22/1 -> Mux2/2
  C32/1 -> Mux2/3
  U/1 -> C32/1, C22/1, C12/1
  Mux2/1 -> U(E)/1

== system Working_TASS2_Fossen/Tgg/Select ci3 ==
  U : Inport  OutDataType=sfix(16)  OutScaling=2^0
  C11 : Fcn  Expr=u[3]
  C12 : Fcn  Expr=u[6]
  C13 : Fcn  Expr=u[9]
  Mux2 : Mux  Inputs=3
  U(E) : Outport  OutDataType=sfix(16)  OutScaling=2^0
  wires:
  Mux2/1 -> U(E)/1
  U/1 -> C13/1, C11/1, C12/1
  C13/1 -> Mux2/3
  C12/1 -> Mux2/2
  C11/1 -> Mux2/1

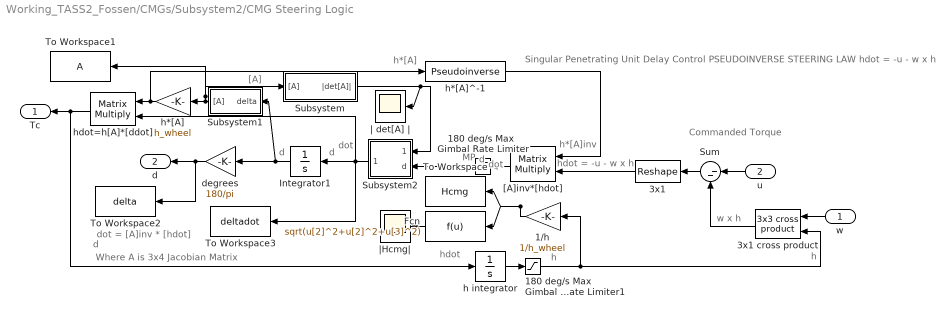
== system Working_TASS2_Fossen/CMGs/Subsystem2/CMG Steering Logic ==
  note: MP
  note: d
  note: dot
  note: d
  note: [A]
  note: h*[A]
  note: h
  note: h*[A]inv
  note: Commanded
      | Torque
  note: Where A is 3x4 Jacobian Matrix
  note: d
  note: dot = [A]inv * [hdot]
  note: Singular Penetrating Unit Delay Control
      | PSEUDOINVERSE STEERING LAW
      | hdot = -u - w x h
  note: w x h
  note: dot
  note: d
  note: hdot = -u - w x h
  note: h
  note: hdot
  w : Inport  OutDataType=sfix(16)  OutScaling=2^0
  u : Inport  Port=2  OutDataType=sfix(16)  OutScaling=2^0
  1/h : Gain  Gain=1/h_wheel  ParameterDataType=sfix(16)  ParameterScaling=2^0  OutDataType=sfix(16)  OutScaling=2^0
  180 deg/s Max  Gimbal Rate Limiter : Saturate  UpperLimit=pi  LowerLimit=-1
  180 deg/s Max  Gimbal Rate Limiter1 : Saturate  UpperLimit=[h_wheel;2*h_wheel;3*h_wheel]  LowerLimit=-1
  3x1 : Reshape  OutputDimensionality=Customize  OutputDimensions=[3,1]
  3x1 cross product : aerospace/Axes Transformations/3x3 cross product  SystemSampleTime=-1
  Fcn : Fcn  Expr=sqrt(u[2]^2+u[2]^2+u[3]^2)
  Integrator1 : Integrator  InitialCondition=Gimbal0
  Subsystem : Subsystem
      mask Display: disp('det[A]')
  Subsystem1 : Subsystem
      mask Display: disp('[A] Matrix')
  Subsystem2 : Subsystem
      mask Display: disp('SPUD')
  Sum : Sum  Inputs=|--  OutDataType=sfix(16)  OutScaling=2^0  SaturateOnIntegerOverflow=on
  To Workspace : ToWorkspace  VariableName=Hcmg  SampleTime=-1  SaveFormat=Array
  To Workspace1 : ToWorkspace  VariableName=A  SampleTime=-1  SaveFormat=Array
  To Workspace2 : ToWorkspace  VariableName=delta  SampleTime=-1  SaveFormat=Array
  To Workspace3 : ToWorkspace  VariableName=deltadot  SampleTime=-1  SaveFormat=Array
  "[A]inv*[hdot]" : Product  Multiplication=Matrix(*)  OutDataType=sfix(16)  OutScaling=2^0  SaturateOnIntegerOverflow=on  OutDataTypeStr=Inherit: Same as first input
  degrees : Gain  Gain=180/pi  ParameterDataType=sfix(16)  ParameterScaling=2^0  OutDataType=sfix(16)  OutScaling=2^0
  h integrator : Integrator
  h*[A] : Gain  Gain=h_wheel  ParameterDataType=sfix(16)  ParameterScaling=2^0  OutDataType=sfix(16)  OutScaling=2^0
  h*[A]^-1 : dspinverses/Pseudoinverse  wanterr=off
  hdot=h[A]*[ddot] : Product  Multiplication=Matrix(*)  OutDataType=sfix(16)  OutScaling=2^0  SaturateOnIntegerOverflow=on  OutDataTypeStr=Inherit: Same as first input
  | det[A] | : Scope
      settings: TimeRange=30  YMin=-1  YMax=1  SaveName=ScopeData9
  |Hcmg| : Scope
      settings: TimeRange=30  YMin=0  YMax=3.5  SaveName=ScopeData5
  Tc : Outport  OutDataType=sfix(16)  OutScaling=2^0
  d : Outport  Port=2  OutDataType=sfix(16)  OutScaling=2^0
  wires:
  180 deg/s Max  Gimbal Rate Limiter/1 -> Subsystem2/2(d)
  3x1 cross product/1 -> Sum/2
  180 deg/s Max  Gimbal Rate Limiter1/1 -> 1/h/1, 3x1 cross product/2
  Subsystem2/1(DeltaDot) -> To Workspace3/1, hdot=h[A]*[ddot]/2, Integrator1/1
  degrees/1 -> To Workspace2/1, d/1
  Integrator1/1 -> degrees/1, Subsystem1/1(delta)
  Subsystem1/1("[A]") -> To Workspace1/1, Subsystem/1("[A]"), h*[A]/1
  Fcn/1 -> |Hcmg|/1
  "[A]inv*[hdot]"/1 -> 180 deg/s Max  Gimbal Rate Limiter/1
  Subsystem/1(|det[A]|) -> Subsystem2/1(|det[A]|), | det[A] |/1
  1/h/1 -> To Workspace/1, Fcn/1
  3x1/1 -> "[A]inv*[hdot]"/2
  h*[A]/1 -> h*[A]^-1/1, hdot=h[A]*[ddot]/1
  hdot=h[A]*[ddot]/1 -> h integrator/1, Tc/1
  h*[A]^-1/1 -> "[A]inv*[hdot]"/1
  u/1 -> Sum/1
  Sum/1 -> 3x1/1
  w/1 -> 3x1 cross product/1
  h integrator/1 -> 180 deg/s Max  Gimbal Rate Limiter1/1

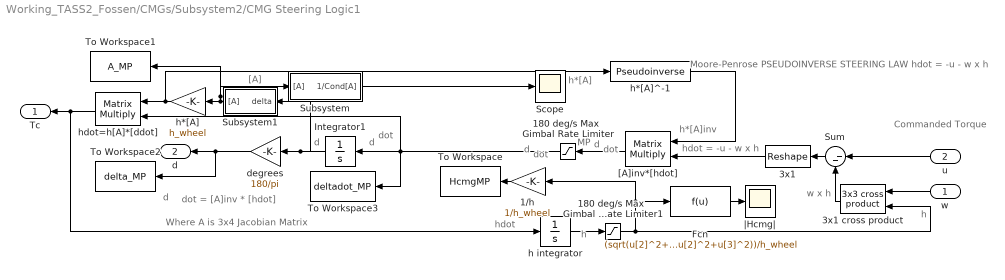
== system Working_TASS2_Fossen/CMGs/Subsystem2/CMG Steering Logic1 ==
  note: hdot
  note: h
  note: hdot = -u - w x h
  note: d
  note: dot
  note: w x h
  note: Moore-Penrose
      | PSEUDOINVERSE STEERING LAW
      | hdot = -u - w x h
  note: dot = [A]inv * [hdot]
  note: d
  note: Where A is 3x4 Jacobian Matrix
  note: Commanded
      | Torque
  note: h*[A]inv
  note: d
  note: dot
  note: h
  note: h*[A]
  note: [A]
  note: d
  note: dot
  note: d
  note: MP
  w : Inport  OutDataType=sfix(16)  OutScaling=2^0
  u : Inport  Port=2  OutDataType=sfix(16)  OutScaling=2^0
  1/h : Gain  Gain=1/h_wheel  ParameterDataType=sfix(16)  ParameterScaling=2^0  OutDataType=sfix(16)  OutScaling=2^0
  180 deg/s Max  Gimbal Rate Limiter : Saturate  UpperLimit=pi  LowerLimit=-1
  180 deg/s Max  Gimbal Rate Limiter1 : Saturate  UpperLimit=[h_wheel;2*h_wheel;3*h_wheel]  LowerLimit=-1
  3x1 : Reshape  OutputDimensionality=Customize  OutputDimensions=[3,1]
  3x1 cross product : aerospace/Axes Transformations/3x3 cross product  SystemSampleTime=-1
  Fcn : Fcn  Expr=(sqrt(u[2]^2+u[2]^2+u[3]^2))/h_wheel
  Integrator1 : Integrator  InitialCondition=Gimbal0
  Scope : Scope
      settings: TimeRange=50  YMin=0  YMax=0.25  SaveName=ScopeData4
  Subsystem : Subsystem
      mask Display: disp('1/Cond[A]')
  Subsystem1 : Subsystem
      mask Display: disp('[A] Matrix')
  Sum : Sum  Inputs=|--  OutDataType=sfix(16)  OutScaling=2^0  SaturateOnIntegerOverflow=on
  To Workspace : ToWorkspace  VariableName=HcmgMP  SampleTime=-1  SaveFormat=Array
  To Workspace1 : ToWorkspace  VariableName=A_MP  SampleTime=-1  SaveFormat=Array
  To Workspace2 : ToWorkspace  VariableName=delta_MP  SampleTime=-1  SaveFormat=Array
  To Workspace3 : ToWorkspace  VariableName=deltadot_MP  SampleTime=-1  SaveFormat=Array
  "[A]inv*[hdot]" : Product  Multiplication=Matrix(*)  OutDataType=sfix(16)  OutScaling=2^0  SaturateOnIntegerOverflow=on  OutDataTypeStr=Inherit: Same as first input
  degrees : Gain  Gain=180/pi  ParameterDataType=sfix(16)  ParameterScaling=2^0  OutDataType=sfix(16)  OutScaling=2^0
  h integrator : Integrator
  h*[A] : Gain  Gain=h_wheel  ParameterDataType=sfix(16)  ParameterScaling=2^0  OutDataType=sfix(16)  OutScaling=2^0
  h*[A]^-1 : dspinverses/Pseudoinverse  wanterr=off
  hdot=h[A]*[ddot] : Product  Multiplication=Matrix(*)  OutDataType=sfix(16)  OutScaling=2^0  SaturateOnIntegerOverflow=on  OutDataTypeStr=Inherit: Same as first input
  |Hcmg| : Scope
      settings: TimeRange=60  YMin=0  YMax=0.9  SaveName=ScopeData5
  Tc : Outport  OutDataType=sfix(16)  OutScaling=2^0
  d : Outport  Port=2  OutDataType=sfix(16)  OutScaling=2^0
  wires:
  1/h/1 -> To Workspace/1
  h integrator/1 -> 180 deg/s Max  Gimbal Rate Limiter1/1
  3x1 cross product/1 -> Sum/2
  w/1 -> 3x1 cross product/1
  Sum/1 -> 3x1/1
  u/1 -> Sum/1
  h*[A]^-1/1 -> "[A]inv*[hdot]"/1
  hdot=h[A]*[ddot]/1 -> Tc/1, h integrator/1
  h*[A]/1 -> hdot=h[A]*[ddot]/1, h*[A]^-1/1
  3x1/1 -> "[A]inv*[hdot]"/2
  180 deg/s Max  Gimbal Rate Limiter1/1 -> Fcn/1, 1/h/1, 3x1 cross product/2
  Subsystem/1(1/Cond[A]) -> Scope/1
  "[A]inv*[hdot]"/1 -> 180 deg/s Max  Gimbal Rate Limiter/1
  Fcn/1 -> |Hcmg|/1
  Subsystem1/1("[A]") -> h*[A]/1, Subsystem/1("[A]"), To Workspace1/1
  Integrator1/1 -> degrees/1, Subsystem1/1(delta)
  degrees/1 -> d/1, To Workspace2/1
  180 deg/s Max  Gimbal Rate Limiter/1 -> Integrator1/1, hdot=h[A]*[ddot]/2, To Workspace3/1

== system Working_TASS2_Fossen/CMGs/Subsystem2/CMG Steering Logic/Subsystem ==
  "[A]" : Inport  OutDataType=sfix(16)  OutScaling=2^0
  | det[A] | : MATLABFcn  MATLABFcn=abs(det(u(:,1:3)))
  |det[A]| : Outport  OutDataType=sfix(16)  OutScaling=2^0
  wires:
  | det[A] |/1 -> |det[A]|/1
  "[A]"/1 -> | det[A] |/1

== system Working_TASS2_Fossen/CMGs/Subsystem2/CMG Steering Logic/Subsystem1 ==
  delta : Inport  OutDataType=sfix(16)  OutScaling=2^0
  3x4 : Reshape  OutputDimensionality=Customize  OutputDimensions=[3,4]
  "[A] Matrix" : MATLABFcn  MATLABFcn="[ -cos(beta(1))*cos(u(1)),  sin(u(2)), cos(beta(3))*cos(u(3)), 0   ;  -sin(u(1)),  -cos(beta(2))*cos(u(2)),  sin(u(3)),   0;  sin(beta(1))*cos(u(1)),  sin(beta(2))*cos(u(2)),  sin(beta(3))*cos(u(3)),   0  ]"
  "[A]" : Outport  OutDataType=sfix(16)  OutScaling=2^0
  wires:
  3x4/1 -> "[A]"/1
  "[A] Matrix"/1 -> 3x4/1
  delta/1 -> "[A] Matrix"/1

== system Working_TASS2_Fossen/CMGs/Subsystem2/CMG Steering Logic/Subsystem2 ==
  note: dot
  note: Engage SPUD
      | DESIGN
      | PARAMETER
  note: dot
  note: d
  |det[A]| : Inport  OutDataType=sfix(16)  OutScaling=2^0
  d : Inport  Port=2  OutDataType=sfix(16)  OutScaling=2^0
  Clock : Clock
      settings: Decimation=10
  Integer Delay : simulink/Discrete/Integer Delay  vinit=0.0  samptime=-1  NumDelays=1
  Switch1 : Switch  Threshold=SPUDengage
  Switch2 : Switch  Threshold=SlewTime+3*DeltaT
  DeltaDot : Outport  OutDataType=sfix(16)  OutScaling=2^0
  wires:
  Switch1/1 -> Switch2/1, DeltaDot/1
  |det[A]|/1 -> Switch1/2
  d/1 -> Switch2/3, Switch1/1
  Integer Delay/1 -> Switch1/3
  Switch2/1 -> Integer Delay/1
  Clock/1 -> Switch2/2

== system Working_TASS2_Fossen/CMGs/Subsystem2/CMG Steering Logic1/Subsystem ==
  "[A]" : Inport  OutDataType=sfix(16)  OutScaling=2^0
  Divide : Product  Inputs=*/  OutDataType=sfix(16)  OutScaling=2^-10
  max (SVD[A]) : MATLABFcn  MATLABFcn=max(svd(u))
  min (SVD[A]) : MATLABFcn  MATLABFcn=min(svd(u))
  1/Cond[A] : Outport  OutDataType=sfix(16)  OutScaling=2^0
  wires:
  "[A]"/1 -> min (SVD[A])/1, max (SVD[A])/1
  min (SVD[A])/1 -> Divide/1
  max (SVD[A])/1 -> Divide/2
  Divide/1 -> 1/Cond[A]/1

== system Working_TASS2_Fossen/CMGs/Subsystem2/CMG Steering Logic1/Subsystem1 ==
  delta : Inport  OutDataType=sfix(16)  OutScaling=2^0
  3x4 : Reshape  OutputDimensionality=Customize  OutputDimensions=[3,4]
  "[A] Matrix" : MATLABFcn  MATLABFcn="[ -cos(beta(1))*cos(u(1)),  sin(u(2)), cos(beta(3))*cos(u(3)), 0   ;  -sin(u(1)),  -cos(beta(2))*cos(u(2)),  sin(u(3)),   0;  sin(beta(1))*cos(u(1)),  sin(beta(2))*cos(u(2)),  sin(beta(3))*cos(u(3)),   0  ]"
  "[A]" : Outport  OutDataType=sfix(16)  OutScaling=2^0
  wires:
  delta/1 -> "[A] Matrix"/1
  "[A] Matrix"/1 -> 3x4/1
  3x4/1 -> "[A]"/1
